simulink model "sampleModel1751"  (R2023a)
settings: Solver=VariableStepAuto  StartTime=0.0  StopTime=10.0  RelTol=1e-3
libraries: hdlsllib x2, simulink x1
settings Model: Creator=user1  LastModifiedBy=user1

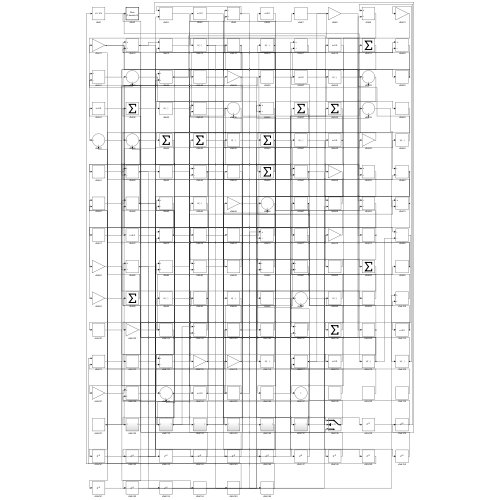
[thumbnail: Simulink's stored preview of the top-level diagram]
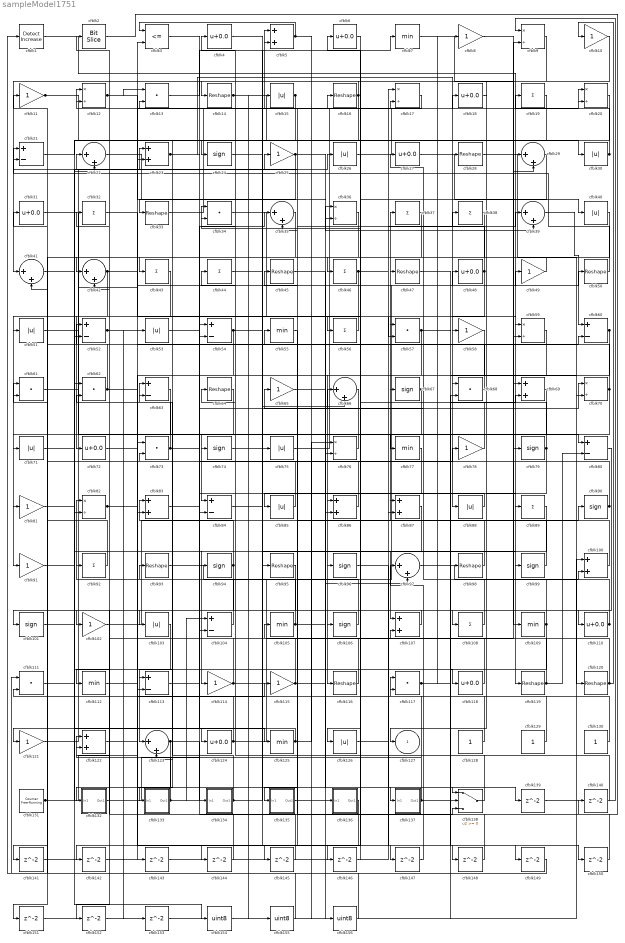
== system sampleModel1751 ==
  cfblk1 : simulink/Logic and Bit Operations/Detect Increase  vinit=0.0  OutDataTypeStr=boolean
      settings: LibrarySourceBlock=|
      | hdlsllib/Logic and Bit
      | Operations/Detect
      | Increase
  cfblk{8,10..11,25,49,58,65,78,81,91,102,114..115,121} (14 alike) : Gain
  cfblk{5,23,69,83,86..87,100,107,122} (9 alike) : Sum
  cfblk{24,67,74,79,90,94,96,99,101,106} (10 alike) : Signum
  cfblk{15,26,30,40,51,53,71,75,85,88,103,126} (12 alike) : Abs  SaturateOnIntegerOverflow=off
  cfblk{21,52,54,60,63,80,84,104,113} (9 alike) : Sum  Inputs=+-
  cfblk{7,55,77,105,109,112,125} (7 alike) : MinMax
  cfblk{19,32,37..38,43..44,46,56,89,92,108} (11 alike) : Sum  Inputs=+
  cfblk{4,6,18,27,31,48,72,110,118,124} (10 alike) : Bias  Bias=0.0  SaturateOnIntegerOverflow=off
  cfblk{13,34,57,61..62,68,73,111,117} (9 alike) : DotProduct  OutDataTypeStr=Inherit: Inherit via internal rule
  cfblk{14,16,28,33,45,47,50,64,93,95,98,116,119..120} (14 alike) : Reshape
  cfblk{9,12,17,20,36,59,70,76,82} (9 alike) : Product  Inputs=*/  RndMeth=Zero  SaturateOnIntegerOverflow=on
  cfblk{22,29,35,39,41..42,66,97,123} (9 alike) : Sum  Inputs=|++
  cfblk128 : Constant  SampleTime=-1
  cfblk129 : Constant  SampleTime=-1
  cfblk130 : Constant  SampleTime=-1
  cfblk131 : hdlsllib/Sources/Counter Free-Running  NumBits=16  tsamp=-1
  cfblk132 : Subsystem
      settings: LibrarySourceBlock=|
      | hdlsllib/Ports &
      | Subsystems/Subsystem
  cfblk133 : Subsystem
      settings: LibrarySourceBlock=|
      | hdlsllib/Ports &
      | Subsystems/Subsystem
  cfblk134 : Subsystem
      settings: LibrarySourceBlock=|
      | hdlsllib/Ports &
      | Subsystems/Subsystem
  cfblk135 : Subsystem
      settings: LibrarySourceBlock=|
      | hdlsllib/Ports &
      | Subsystems/Subsystem
  cfblk136 : Subsystem
      settings: LibrarySourceBlock=|
      | hdlsllib/Ports &
      | Subsystems/Subsystem
  cfblk137 : Subsystem
      settings: LibrarySourceBlock=|
      | hdlsllib/Ports &
      | Subsystems/Subsystem
  cfblk138 : Switch  SaturateOnIntegerOverflow=off  InputSameDT=off
  cfblk{139..153} (15 alike) : Delay  SampleTime=1
  cfblk154 : DataTypeConversion  OutDataTypeStr=uint8  SaturateOnIntegerOverflow=off  RndMeth=Floor
  cfblk155 : DataTypeConversion  OutDataTypeStr=uint8  SaturateOnIntegerOverflow=off  RndMeth=Floor
  cfblk156 : DataTypeConversion  OutDataTypeStr=uint8  SaturateOnIntegerOverflow=off  RndMeth=Floor
  cfblk2 : hdlsllib/Logic and Bit Operations/Bit Slice  lidx=7  ridx=0
  cfblk3 : RelationalOperator  Operator=<=  OutDataTypeStr=boolean  InputSameDT=off
  cfblk127 : Outport  VectorParamsAs1DForOutWhenUnconnected=off
  wires:
  cfblk16/1 -> cfblk14/1, cfblk84/2
  cfblk121/1 -> cfblk23/1
  cfblk46/1 -> cfblk91/1, cfblk38/1
  cfblk93/1 -> cfblk16/1
  cfblk64/1 -> cfblk81/1
  cfblk23/1 -> cfblk88/1, cfblk77/1
  cfblk1/1 -> cfblk119/1
  cfblk48/1 -> cfblk58/1, cfblk21/2
  cfblk88/1 -> cfblk85/1
  cfblk4/1 -> cfblk95/1
  cfblk51/1 -> cfblk25/1
  cfblk92/1 -> cfblk61/1
  cfblk18/1 -> cfblk127/1
  cfblk107/1 -> cfblk102/1
  cfblk15/1 -> cfblk33/1, cfblk52/2
  cfblk122/1 -> cfblk53/1
  cfblk27/1 -> cfblk40/1
  cfblk42/1 -> cfblk72/1, cfblk57/2
  cfblk58/1 -> cfblk116/1
  cfblk75/1 -> cfblk17/2
  cfblk24/1 -> cfblk7/1
  cfblk31/1 -> cfblk84/1
  cfblk12/1 -> cfblk13/1, cfblk36/2
  cfblk133/1(Out1) -> cfblk32/1, cfblk35/1, cfblk104/1, cfblk138/3
  cfblk89/1 -> cfblk107/1
  cfblk52/1 -> cfblk47/1, cfblk153/1
  cfblk10/1 -> cfblk41/1
  cfblk5/1 -> cfblk3/1, cfblk156/1
  cfblk87/1 -> cfblk114/1
  cfblk34/1 -> cfblk59/1
  cfblk35/1 -> cfblk42/1
  cfblk98/1 -> cfblk37/1
  cfblk97/1 -> cfblk100/2
  cfblk84/1 -> cfblk66/2
  cfblk116/1 -> cfblk44/1
  cfblk49/1 -> cfblk43/1
  cfblk61/1 -> cfblk3/2
  cfblk83/1 -> cfblk78/1
  cfblk30/1 -> cfblk19/1, cfblk24/1
  cfblk13/1 -> cfblk5/1
  cfblk109/1 -> cfblk52/1, cfblk138/2
  cfblk95/1 -> cfblk112/1
  cfblk124/1 -> cfblk48/1, cfblk41/2
  cfblk118/1 -> cfblk55/1
  cfblk76/1 -> cfblk74/1
  cfblk66/1 -> cfblk106/1
  cfblk104/1 -> cfblk82/1
  cfblk41/1 -> cfblk94/1
  cfblk103/1 -> cfblk123/1
  cfblk65/1 -> cfblk49/1
  cfblk43/1 -> cfblk82/2
  cfblk71/1 -> cfblk26/1
  cfblk38/1 -> cfblk71/1
  cfblk106/1 -> cfblk45/1
  cfblk94/1 -> cfblk83/1, cfblk132/1(In1)
  cfblk132/1(Out1) -> cfblk54/1
  cfblk56/1 -> cfblk51/1
  cfblk100/1 -> cfblk87/1
  cfblk80/1 -> cfblk110/1
  cfblk29/1 -> cfblk56/1
  cfblk28/1 -> cfblk120/1
  cfblk14/1 -> cfblk28/1, cfblk155/1
  cfblk62/1 -> cfblk31/1, cfblk20/2, cfblk139/1
  cfblk113/1 -> cfblk70/1
  cfblk57/1 -> cfblk96/1, cfblk150/1
  cfblk81/1 -> cfblk124/1
  cfblk33/1 -> cfblk5/2
  cfblk47/1 -> cfblk70/2
  cfblk85/1 -> cfblk61/2
  cfblk26/1 -> cfblk20/1
  cfblk68/1 -> cfblk27/1
  cfblk137/1(Out1) -> cfblk122/1, cfblk117/2, cfblk69/2
  cfblk99/1 -> cfblk15/1
  cfblk120/1 -> cfblk10/1, cfblk42/2
  cfblk44/1 -> cfblk138/1
  cfblk59/1 -> cfblk135/1(In1)
  cfblk79/1 -> cfblk108/1, cfblk12/2
  cfblk128/1 -> cfblk64/1
  cfblk101/1 -> cfblk118/1
  cfblk39/1 -> cfblk60/1
  cfblk70/1 -> cfblk34/1, cfblk104/2
  cfblk9/1 -> cfblk68/1
  cfblk32/1 -> cfblk59/2
  cfblk6/1 -> cfblk86/1
  cfblk19/1 -> cfblk29/1
  cfblk86/1 -> cfblk22/1
  cfblk138/1 -> cfblk4/1
  cfblk119/1 -> cfblk105/1, cfblk80/2, cfblk93/1
  cfblk60/1 -> cfblk133/1(In1), cfblk76/2
  cfblk134/1(Out1) -> cfblk18/1, cfblk50/1, cfblk63/1
  cfblk105/1 -> cfblk97/2, cfblk63/2
  cfblk7/1 -> cfblk29/2
  cfblk22/1 -> cfblk75/1
  cfblk110/1 -> cfblk67/1, cfblk101/1
  cfblk25/1 -> cfblk113/1, cfblk39/2
  cfblk17/1 -> cfblk13/2
  cfblk21/1 -> cfblk30/1
  cfblk67/1 -> cfblk113/2, cfblk141/1
  cfblk73/1 -> cfblk2/1, cfblk125/1
  cfblk102/1 -> cfblk90/1
  cfblk36/1 -> cfblk123/2
  cfblk135/1(Out1) -> cfblk136/1(In1)
  cfblk90/1 -> cfblk73/2, cfblk6/1
  cfblk112/1 -> cfblk57/1
  cfblk20/1 -> cfblk54/2
  cfblk123/1 -> cfblk134/1(In1), cfblk152/1
  cfblk53/1 -> cfblk89/1
  cfblk114/1 -> cfblk9/2, cfblk92/1
  cfblk125/1 -> cfblk121/1, cfblk76/1
  cfblk115/1 -> cfblk12/1, cfblk60/2
  cfblk37/1 -> cfblk103/1
  cfblk78/1 -> cfblk34/2
  cfblk40/1 -> cfblk46/1
  cfblk3/1 -> cfblk80/1
  cfblk69/1 -> cfblk126/1
  cfblk11/1 -> cfblk69/1, cfblk109/1
  cfblk54/1 -> cfblk83/2, cfblk99/1
  cfblk126/1 -> cfblk39/1
  cfblk50/1 -> cfblk21/1
  cfblk129/1 -> cfblk117/1
  cfblk130/1 -> cfblk11/1
  cfblk45/1 -> cfblk137/1(In1)
  cfblk91/1 -> cfblk62/1
  cfblk8/1 -> cfblk79/1
  cfblk82/1 -> cfblk143/1, cfblk144/1
  cfblk108/1 -> cfblk65/1
  cfblk131/1 -> cfblk115/1, cfblk22/2
  cfblk117/1 -> cfblk98/1, cfblk8/1
  cfblk139/1 -> cfblk9/1
  cfblk2/1 -> cfblk140/1
  cfblk140/1 -> cfblk97/1
  cfblk141/1 -> cfblk23/2
  cfblk136/1(Out1) -> cfblk142/1
  cfblk142/1 -> cfblk73/1
  cfblk143/1 -> cfblk87/2
  cfblk144/1 -> cfblk62/2
  cfblk55/1 -> cfblk145/1
  cfblk145/1 -> cfblk122/2
  cfblk77/1 -> cfblk146/1
  cfblk146/1 -> cfblk66/1
  cfblk74/1 -> cfblk147/1
  cfblk147/1 -> cfblk107/2
  cfblk72/1 -> cfblk148/1
  cfblk148/1 -> cfblk17/1
  cfblk96/1 -> cfblk149/1
  cfblk149/1 -> cfblk1/1
  cfblk150/1 -> cfblk35/2
  cfblk63/1 -> cfblk151/1
  cfblk151/1 -> cfblk68/2
  cfblk152/1 -> cfblk86/2
  cfblk153/1 -> cfblk100/1
  cfblk111/1 -> cfblk154/1
  cfblk154/1 -> cfblk36/1
  cfblk155/1 -> cfblk111/1
  cfblk156/1 -> cfblk111/2

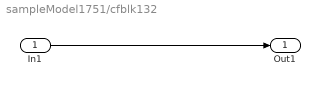
== system sampleModel1751/cfblk132 ==
  In1 : Inport
  Out1 : Outport
  wires:
  In1/1 -> Out1/1

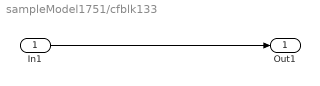
== system sampleModel1751/cfblk133 ==
  In1 : Inport
  Out1 : Outport
  wires:
  In1/1 -> Out1/1

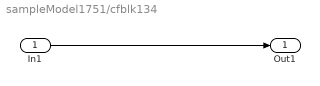
== system sampleModel1751/cfblk134 ==
  In1 : Inport
  Out1 : Outport
  wires:
  In1/1 -> Out1/1

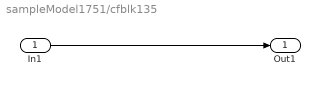
== system sampleModel1751/cfblk135 ==
  In1 : Inport
  Out1 : Outport
  wires:
  In1/1 -> Out1/1

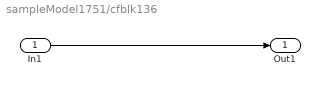
== system sampleModel1751/cfblk136 ==
  In1 : Inport
  Out1 : Outport
  wires:
  In1/1 -> Out1/1

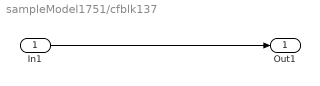
== system sampleModel1751/cfblk137 ==
  In1 : Inport
  Out1 : Outport
  wires:
  In1/1 -> Out1/1
